simulink model "vasastaden_sort"  (Simulink 5.0)
settings: Solver=FixedStepDiscrete  SolverMode=SingleTasking  StartTime=0  StopTime=Q  FixedStep=1  RelTol=1e-3
values from neighbouring files (symbols this model uses):
  andpt = 1/3    (= 0.333333333333)    [constants_trafik.m]
  andt = 0.1    [constants_trafik.m]
  baseflow = str2num(get(HH, 'String'))    [inputs.m]
  baseflow2 = 0    [areas2.m]
  delayinit = [zeros(1,nr_ex_H2O)]    [constants_trafik.m]
  fast = 0.7    [constants_trafik.m]
  fkmday = in_fkmday    [areas.m]
  fkmday2 = 32067    [areas2.m]
  init_init = 4*3600    (= 14400)    [areas.m]
  init_time = 5    [areas.m]
  K2 = 0.03    [areas2.m]
  nhv = in_nhv/100    [areas.m]
  nhv2 = 5/100    (= 0.05)    [areas2.m]
  nr_ex_H2O = totnr-1    (= 20)    [Prep.m]
  numberOfPersons = in_numberOfPersons    [Prep.m]
  numberOfPersons2 = 5115    [areas2.m]
  othera = in_otherarea    [areas.m]
  othera2 = 42282    [areas2.m]
  othermax = drydepmax*othera    [constants_trafik.m]
  othermax2 = drydepmax*othera2    [areas2.m]
  redu = 0.8    [areas.m]
  roada = in_roads    [areas.m]
  roada2 = 95962    [areas2.m]
  roadaccmax = dryper*24*sph*fast*(p_tyrewear+p_roadwear+p_exhaust+p_breakwear+p_drydep+p_corrZn+p_oildischarge+p_catalyst)    [constants_trafik.m]
  roadaccmax2 = dryper*24*sph*fast*(p_tyrewear2+p_roadwear2+p_exhaust2+p_breakwear2+p_drydep2+p_corrZn2+p_oildischarge2+p_catalyst2)    [areas2.m]
  roadkm = 67e9    (= 67000000000)    [constants_trafik.m]
  roadrunpart = 1    [constants_trafik.m]
  roadwear = 130000    [constants_trafik.m]
  roadZna = in_part_roadZna/100*roada    [areas.m]
  roadZna2 = 2/100*roada2    (= 1919.24)    [areas2.m]
  roofa = in_roofs    [areas.m]
  roofa2 = 92958    [areas2.m]
  RoofCua = in_part_roofCua/100*roofa/cos(15*pi/180)    [areas.m]
  RoofCua2 = 6.9/100*roofa2/cos(15*pi/180)    [areas2.m]
  roofmax = (Znroofmax*RoofZna+Curoofmax*RoofCua)*roofrunpart+drydepmax*roofa    [constants_trafik.m]
  roofmax2 = (Znroofmax*RoofZna2+Curoofmax*RoofCua2)*roofrunpart+drydepmax*roofa2    [areas2.m]
  roofrunpart = 0.7    [constants_trafik.m]
  RoofZna = in_part_roofZna/100*roofa/cos(15*pi/180)    [areas.m]
  RoofZna2 = 6.4/100*roofa2/cos(15*pi/180)    [areas2.m]
  sec_per_ts = in_sec_per_ts    [Prep.m]
  sph = 3600/sec_per_ts    [Prep.m]
  tota = in_tota    [areas.m]
  totnr = 21    [Prep.m]
  tyrewear = 9000    [constants_trafik.m]
  wetdep = [sum(s_wetdep(:,i))]*tota*trans1    [polldistr_gr.m]
  yearly_rain = 1    [Callback_simulate.m]    (also in SEWSYS_fig.m)
undefined symbols (not defined in the file or in its folder): BDT, BODofVS, brakep, catalystp, Curoofp, Drainage, drydep, exhp, Faeces, Industry, K, K2r, oilp, ProcSS_bio, ProcSS_chem, ProcSS_presed, ProcSS_sand, ProcSS_screen, roadp, sani, spBiooxidBod, spBiored, spCcontent, spChemFe, spChemicalPart, spCODBOD, spDenSS, spHeavym, spHjust, spN2ONpurEmitted, spNemitted, spNitrif, spNpur, spOcontent, spPBound, spPout, spPout1, spVSofSS, SSred_bio, SSred_chem, SSred_presed, SSred_sand, SSred_screen, SStoWater, stormw, tyrep, Urine, VSofSS_sand, VSofSS_screen, Znroofp
libraries: SEWSYS_library x1
(part 3 of 3)

== system vasastaden_sort/Separate Sewer System  (1245)/Stormwater/Storm water/Runoff/Subsystem1/if u>0 then u else 1 ==
  note: if u<=0, 0, else u, end
  in_1 : Inport
  Constant : Constant  Value=0
  Switch : Switch  SaturateOnIntegerOverflow=on  InputSameDT=on
  inv. : Fcn  Expr=u
  neg : Gain  Gain=-1  SaturateOnIntegerOverflow=on
  out_1 : Outport  InitialOutput=0
  wires:
  in_1/1 -> inv./1, neg/1
  inv./1 -> Switch/3
  neg/1 -> Switch/2
  Constant/1 -> Switch/1
  Switch/1 -> out_1/1

== system vasastaden_sort/Sewage plant/Biological stage/Predenitri- fication/Nitrification/ denitrification/N-org to NH4/if u>0 then 1/u else 0 ==
  note: if u<=0, 0, else 1/u, end
  in_1 : Inport  Orientation=left
  Constant : Constant  Orientation=left  Value=0
  Constant1 : Constant  Orientation=left
  Switch : Switch  Orientation=left  SaturateOnIntegerOverflow=on  InputSameDT=on
  Switch1 : Switch  Orientation=left  SaturateOnIntegerOverflow=on  InputSameDT=on
  inv. : Fcn  Orientation=left  Expr=1/u
  neg : Gain  Orientation=left  Gain=-1  SaturateOnIntegerOverflow=on
  out_1 : Outport  Orientation=left  InitialOutput=0
  wires:
  Constant1/1 -> Switch1/1
  in_1/1 -> Switch1/3, neg/1
  neg/1 -> Switch1/2, Switch/2
  Switch1/1 -> inv./1
  Switch/1 -> out_1/1
  inv./1 -> Switch/3
  Constant/1 -> Switch/1

== system vasastaden_sort/Separate Sewer System  (36)/Stormwater/Storm water/Add pollutants in rain/Initial loss/Count zeros/Counter1 ==
  Enable : EnablePort  StatesWhenEnabling=reset
  Constant7 : Constant
  Discrete-Time Integrator : DiscreteIntegrator  InitialCondition=1
  Out1 : Outport  InitialOutput=0
  wires:
  Discrete-Time Integrator/1 -> Out1/1
  Constant7/1 -> Discrete-Time Integrator/1

== system vasastaden_sort/Separate Sewer System  (36)/Stormwater/Storm water/Rain -> Stormwater/road surfaces/pollutants on roads/brake wear ==
  note: [ug/fkm]
  Product : Product  Inputs=*/  SaturateOnIntegerOverflow=on  InputSameDT=on
  Product1 : Product  SaturateOnIntegerOverflow=on  InputSameDT=on
  fordonskm/day : Constant  Value=fkmday2
  pollutants from brakes : Constant  Value=brakep
  timesteps/day : Constant  Value=24*sph
  "pollutants [ug) " : Outport
  wires:
  Product1/1 -> "pollutants [ug) "/1
  pollutants from brakes/1 -> Product1/2
  fordonskm/day/1 -> Product/1
  timesteps/day/1 -> Product/2
  Product/1 -> Product1/1

== system vasastaden_sort/Separate Sewer System  (36)/Stormwater/Storm water/Rain -> Stormwater/road surfaces/pollutants on roads/catalyst ==
  note: [ug/fkm]
  Product : Product  Inputs=*/  SaturateOnIntegerOverflow=on  InputSameDT=on
  Product1 : Product  SaturateOnIntegerOverflow=on  InputSameDT=on
  fordonskm/day : Constant  Value=fkmday2
  pollutants from catalysts : Constant  Value=catalystp
  timesteps/day : Constant  Value=24*sph
  "pollutants [ug) " : Outport
  wires:
  Product1/1 -> "pollutants [ug) "/1
  pollutants from catalysts/1 -> Product1/2
  fordonskm/day/1 -> Product/1
  timesteps/day/1 -> Product/2
  Product/1 -> Product1/1

== system vasastaden_sort/Separate Sewer System  (36)/Stormwater/Storm water/Rain -> Stormwater/road surfaces/pollutants on roads/corrosion-Zn ==
  Product : Product  SaturateOnIntegerOverflow=on  InputSameDT=on
  area [m2] : Constant  Value=roadZna2
  avrunnen andel : Gain  Gain=roadrunpart  SaturateOnIntegerOverflow=on
  pollutants from  zink surface : Subsystem
  pollutants [ug] : Outport
  wires:
  Product/1 -> pollutants [ug]/1
  pollutants from  zink surface/1("[ug/m2]") -> avrunnen andel/1
  avrunnen andel/1 -> Product/1
  area [m2]/1 -> Product/2

== system vasastaden_sort/Separate Sewer System  (36)/Stormwater/Storm water/Rain -> Stormwater/road surfaces/pollutants on roads/dry deposition ==
  Product : Product  Inputs=*/  SaturateOnIntegerOverflow=on  InputSameDT=on
  Product1 : Product  SaturateOnIntegerOverflow=on  InputSameDT=on
  area m2 : Constant  Orientation=up  Value=roada2
  timesteps/yr : Constant  Value=365*24*sph
  torrdep ug/m2*yr : Constant  Value=drydep
  pollutants [ug] : Outport
  wires:
  timesteps/yr/1 -> Product/2
  torrdep ug/m2*yr/1 -> Product/1
  Product/1 -> Product1/1
  Product1/1 -> pollutants [ug]/1
  area m2/1 -> Product1/2

== system vasastaden_sort/Separate Sewer System  (36)/Stormwater/Storm water/Rain -> Stormwater/road surfaces/pollutants on roads/exhaust ==
  Product : Product  SaturateOnIntegerOverflow=on  InputSameDT=on
  Product1 : Product  Inputs=*/  SaturateOnIntegerOverflow=on  InputSameDT=on
  fordonskm/day : Constant  Value=fkmday2
  pollutant [ug/fkm] : Constant  Value=exhp
  timesteps/day : Constant  Value=24*sph
  pollutant [ug] : Outport
  wires:
  fordonskm/day/1 -> Product1/1
  timesteps/day/1 -> Product1/2
  Product/1 -> pollutant [ug]/1
  pollutant [ug/fkm]/1 -> Product/2
  Product1/1 -> Product/1

== system vasastaden_sort/Separate Sewer System  (36)/Stormwater/Storm water/Rain -> Stormwater/road surfaces/pollutants on roads/oil discharge ==
  note: [ug/fkm]
  Product : Product  Inputs=*/  SaturateOnIntegerOverflow=on  InputSameDT=on
  Product1 : Product  SaturateOnIntegerOverflow=on  InputSameDT=on
  fordonskm/day : Constant  Value=fkmday2
  pollutants from oil : Constant  Value=oilp
  timesteps/day : Constant  Value=24*sph
  "pollutants [ug) " : Outport
  wires:
  Product/1 -> Product1/1
  timesteps/day/1 -> Product/2
  fordonskm/day/1 -> Product/1
  pollutants from oil/1 -> Product1/2
  Product1/1 -> "pollutants [ug) "/1

== system vasastaden_sort/Separate Sewer System  (36)/Stormwater/Storm water/Rain -> Stormwater/road surfaces/pollutants on roads/road wear ==
  note: kilos of road material
      | per time unit
  Fcn : Fcn  Expr=1-u[1]
  Product : Product  Inputs=3  SaturateOnIntegerOverflow=on  InputSameDT=on
  Product1 : Product  Inputs=3  SaturateOnIntegerOverflow=on  InputSameDT=on
  Product2 : Product  SaturateOnIntegerOverflow=on  InputSameDT=on
  Product3 : Product  Inputs=*/  SaturateOnIntegerOverflow=on  InputSameDT=on
  Road wear : Subsystem
  Sum : Sum  Inputs=|++  SaturateOnIntegerOverflow=on  InputSameDT=on
  andel tunga fordon : Constant  Value=nhv2
  fordonskm/day : Constant  Value=fkmday2
  mg->ug : Gain  Gain=1000  SaturateOnIntegerOverflow=on
  "pollutants in road mat. ppm " : Constant  Orientation=up  Value=roadp
  timesteps/day : Constant  Value=24*sph
  pollutants [ug] : Outport
  wires:
  mg->ug/1 -> pollutants [ug]/1
  Road wear/1(vägslitage kg/tfkm) -> Product/1
  Road wear/2(vägslitage kg/pbkm) -> Product1/3
  Sum/1 -> Product2/1
  Product/1 -> Sum/1
  Product1/1 -> Sum/2
  Fcn/1 -> Product1/2
  andel tunga fordon/1 -> Fcn/1, Product/2
  "pollutants in road mat. ppm "/1 -> Product2/2
  Product2/1 -> mg->ug/1
  timesteps/day/1 -> Product3/2
  fordonskm/day/1 -> Product3/1
  Product3/1 -> Product/3, Product1/1

== system vasastaden_sort/Separate Sewer System  (36)/Stormwater/Storm water/Rain -> Stormwater/road surfaces/pollutants on roads/tyre wear ==
  note: [mg]
  note: Kilos of tyre per
      | time unit
  Fcn : Fcn  Expr=1-u[1]
  Gain : Gain  Gain=1000  SaturateOnIntegerOverflow=on
  Product : Product  Inputs=3  SaturateOnIntegerOverflow=on  InputSameDT=on
  Product1 : Product  Inputs=3  SaturateOnIntegerOverflow=on  InputSameDT=on
  Product2 : Product  SaturateOnIntegerOverflow=on  InputSameDT=on
  Product3 : Product  Inputs=*/  SaturateOnIntegerOverflow=on  InputSameDT=on
  Sum : Sum  Inputs=|++  SaturateOnIntegerOverflow=on  InputSameDT=on
  andel tunga fordon : Constant  Value=nhv2
  fordonskm/day : Constant  Value=fkmday2
  pollutants in tyre  [ppm] : Constant  Orientation=up  Value=tyrep
  timesteps/day : Constant  Value=24*sph
  tyre wear : Subsystem
  pollutants [ug] : Outport
  wires:
  Gain/1 -> pollutants [ug]/1
  pollutants in tyre  [ppm]/1 -> Product2/2
  Sum/1 -> Product2/1
  andel tunga fordon/1 -> Product/2, Fcn/1
  Fcn/1 -> Product1/2
  Product1/1 -> Sum/2
  Product/1 -> Sum/1
  Product2/1 -> Gain/1
  tyre wear/1(tyre wear [kg/tfkm]) -> Product/1
  tyre wear/2(tyre wear [kg/pbkm]) -> Product1/3
  timesteps/day/1 -> Product3/2
  fordonskm/day/1 -> Product3/1
  Product3/1 -> Product/3, Product1/1

== system vasastaden_sort/Separate Sewer System  (36)/Stormwater/Storm water/Rain -> Stormwater/roofs/Pollutants on roofs/Corrosion-Cu ==
  Product : Product  SaturateOnIntegerOverflow=on  InputSameDT=on
  Product1 : Product  Inputs=*/  SaturateOnIntegerOverflow=on  InputSameDT=on
  area [m2] : Constant  Value=RoofCua2
  avrunnen andel : Gain  Gain=roofrunpart  SaturateOnIntegerOverflow=on
  g/m2->ug/m2 : Gain  Gain=1000000  SaturateOnIntegerOverflow=on
  pollutants [g/m2*yr] : Constant  Value=Curoofp
  timesteps/yr : Constant  Value=365*24*sph
  pollutants [ug] : Outport
  wires:
  pollutants [g/m2*yr]/1 -> g/m2->ug/m2/1
  Product1/1 -> avrunnen andel/1
  g/m2->ug/m2/1 -> Product1/1
  timesteps/yr/1 -> Product1/2
  area [m2]/1 -> Product/2
  avrunnen andel/1 -> Product/1
  Product/1 -> pollutants [ug]/1

== system vasastaden_sort/Separate Sewer System  (36)/Stormwater/Storm water/Rain -> Stormwater/roofs/Pollutants on roofs/Corrosion-Zn ==
  Product : Product  SaturateOnIntegerOverflow=on  InputSameDT=on
  Product1 : Product  Inputs=*/  SaturateOnIntegerOverflow=on  InputSameDT=on
  area [m2] : Constant  Value=RoofZna2
  avrunnen andel : Gain  Gain=roofrunpart  SaturateOnIntegerOverflow=on
  g/m2->ug/m2 : Gain  Gain=1000000  SaturateOnIntegerOverflow=on
  pollutants [g/m2*yr] : Constant  Value=Znroofp
  timesteps/yr : Constant  Value=365*24*sph
  pollutants [ug] : Outport
  wires:
  Product1/1 -> avrunnen andel/1
  timesteps/yr/1 -> Product1/2
  pollutants [g/m2*yr]/1 -> g/m2->ug/m2/1
  g/m2->ug/m2/1 -> Product1/1
  Product/1 -> pollutants [ug]/1
  avrunnen andel/1 -> Product/1
  area [m2]/1 -> Product/2

== system vasastaden_sort/Separate Sewer System  (36)/Stormwater/Storm water/Rain -> Stormwater/roofs/Pollutants on roofs/dry deposition ==
  Product : Product  Inputs=*/  SaturateOnIntegerOverflow=on  InputSameDT=on
  Product1 : Product  SaturateOnIntegerOverflow=on  InputSameDT=on
  area m2 : Constant  Orientation=up  Value=roofa2
  timesteps/yr : Constant  Value=365*24*sph
  torrdep ug/m2*yr : Constant  Value=drydep
  pollutants [ug] : Outport
  wires:
  timesteps/yr/1 -> Product/2
  torrdep ug/m2*yr/1 -> Product/1
  Product/1 -> Product1/1
  Product1/1 -> pollutants [ug]/1
  area m2/1 -> Product1/2

== system vasastaden_sort/Separate Sewer System  (1245)/Stormwater/Storm water/Add pollutants in rain/Initial loss/Count zeros/Counter1 ==
  Enable : EnablePort  StatesWhenEnabling=reset
  Constant7 : Constant
  Discrete-Time Integrator : DiscreteIntegrator  InitialCondition=1
  Out1 : Outport  InitialOutput=0
  wires:
  Constant7/1 -> Discrete-Time Integrator/1
  Discrete-Time Integrator/1 -> Out1/1

== system vasastaden_sort/Separate Sewer System  (1245)/Stormwater/Storm water/Rain -> Stormwater/road surfaces/pollutants on roads/brake wear ==
  note: [ug/fkm]
  Product : Product  Inputs=*/  SaturateOnIntegerOverflow=on  InputSameDT=on
  Product1 : Product  SaturateOnIntegerOverflow=on  InputSameDT=on
  fordonskm/day : Constant  Value=fkmday
  pollutants from brakes : Constant  Value=brakep
  timesteps/day : Constant  Value=24*sph
  "pollutants [ug) " : Outport
  wires:
  Product/1 -> Product1/1
  timesteps/day/1 -> Product/2
  fordonskm/day/1 -> Product/1
  pollutants from brakes/1 -> Product1/2
  Product1/1 -> "pollutants [ug) "/1

== system vasastaden_sort/Separate Sewer System  (1245)/Stormwater/Storm water/Rain -> Stormwater/road surfaces/pollutants on roads/catalyst ==
  note: [ug/fkm]
  Product : Product  Inputs=*/  SaturateOnIntegerOverflow=on  InputSameDT=on
  Product1 : Product  SaturateOnIntegerOverflow=on  InputSameDT=on
  fordonskm/day : Constant  Value=fkmday
  pollutants from catalysts : Constant  Value=catalystp
  timesteps/day : Constant  Value=24*sph
  "pollutants [ug) " : Outport
  wires:
  Product/1 -> Product1/1
  timesteps/day/1 -> Product/2
  fordonskm/day/1 -> Product/1
  pollutants from catalysts/1 -> Product1/2
  Product1/1 -> "pollutants [ug) "/1

== system vasastaden_sort/Separate Sewer System  (1245)/Stormwater/Storm water/Rain -> Stormwater/road surfaces/pollutants on roads/corrosion-Zn ==
  Product : Product  SaturateOnIntegerOverflow=on  InputSameDT=on
  area [m2] : Constant  Value=roadZna
  avrunnen andel : Gain  Gain=roadrunpart  SaturateOnIntegerOverflow=on
  pollutants from  zink surface : Subsystem
  pollutants [ug] : Outport
  wires:
  area [m2]/1 -> Product/2
  avrunnen andel/1 -> Product/1
  pollutants from  zink surface/1("[ug/m2]") -> avrunnen andel/1
  Product/1 -> pollutants [ug]/1

== system vasastaden_sort/Separate Sewer System  (1245)/Stormwater/Storm water/Rain -> Stormwater/road surfaces/pollutants on roads/dry deposition ==
  Product : Product  Inputs=*/  SaturateOnIntegerOverflow=on  InputSameDT=on
  Product1 : Product  SaturateOnIntegerOverflow=on  InputSameDT=on
  area m2 : Constant  Orientation=up  Value=roada
  timesteps/yr : Constant  Value=365*24*sph
  torrdep ug/m2*yr : Constant  Value=drydep
  pollutants [ug] : Outport
  wires:
  area m2/1 -> Product1/2
  Product1/1 -> pollutants [ug]/1
  Product/1 -> Product1/1
  torrdep ug/m2*yr/1 -> Product/1
  timesteps/yr/1 -> Product/2

== system vasastaden_sort/Separate Sewer System  (1245)/Stormwater/Storm water/Rain -> Stormwater/road surfaces/pollutants on roads/exhaust ==
  Product : Product  SaturateOnIntegerOverflow=on  InputSameDT=on
  Product1 : Product  Inputs=*/  SaturateOnIntegerOverflow=on  InputSameDT=on
  fordonskm/day : Constant  Value=fkmday
  pollutant [ug/fkm] : Constant  Value=exhp
  timesteps/day : Constant  Value=24*sph
  pollutant [ug] : Outport
  wires:
  Product1/1 -> Product/1
  pollutant [ug/fkm]/1 -> Product/2
  Product/1 -> pollutant [ug]/1
  timesteps/day/1 -> Product1/2
  fordonskm/day/1 -> Product1/1

== system vasastaden_sort/Separate Sewer System  (1245)/Stormwater/Storm water/Rain -> Stormwater/road surfaces/pollutants on roads/oil discharge ==
  note: [ug/fkm]
  Product : Product  Inputs=*/  SaturateOnIntegerOverflow=on  InputSameDT=on
  Product1 : Product  SaturateOnIntegerOverflow=on  InputSameDT=on
  fordonskm/day : Constant  Value=fkmday
  pollutants from oil : Constant  Value=oilp
  timesteps/day : Constant  Value=24*sph
  "pollutants [ug) " : Outport
  wires:
  Product1/1 -> "pollutants [ug) "/1
  pollutants from oil/1 -> Product1/2
  fordonskm/day/1 -> Product/1
  timesteps/day/1 -> Product/2
  Product/1 -> Product1/1

== system vasastaden_sort/Separate Sewer System  (1245)/Stormwater/Storm water/Rain -> Stormwater/road surfaces/pollutants on roads/road wear ==
  note: kilos of road material
      | per time unit
  Fcn : Fcn  Expr=1-u[1]
  Product : Product  Inputs=3  SaturateOnIntegerOverflow=on  InputSameDT=on
  Product1 : Product  Inputs=3  SaturateOnIntegerOverflow=on  InputSameDT=on
  Product2 : Product  SaturateOnIntegerOverflow=on  InputSameDT=on
  Product3 : Product  Inputs=*/  SaturateOnIntegerOverflow=on  InputSameDT=on
  Road wear : Subsystem
  Sum : Sum  Inputs=|++  SaturateOnIntegerOverflow=on  InputSameDT=on
  andel tunga fordon : Constant  Value=nhv
  fordonskm/day : Constant  Value=fkmday
  mg->ug : Gain  Gain=1000  SaturateOnIntegerOverflow=on
  "pollutants in road mat. ppm " : Constant  Orientation=up  Value=roadp
  timesteps/day : Constant  Value=24*sph
  pollutants [ug] : Outport
  wires:
  Product3/1 -> Product1/1, Product/3
  fordonskm/day/1 -> Product3/1
  timesteps/day/1 -> Product3/2
  Product2/1 -> mg->ug/1
  "pollutants in road mat. ppm "/1 -> Product2/2
  andel tunga fordon/1 -> Product/2, Fcn/1
  Fcn/1 -> Product1/2
  Product1/1 -> Sum/2
  Product/1 -> Sum/1
  Sum/1 -> Product2/1
  Road wear/2(vägslitage kg/pbkm) -> Product1/3
  Road wear/1(vägslitage kg/tfkm) -> Product/1
  mg->ug/1 -> pollutants [ug]/1

== system vasastaden_sort/Separate Sewer System  (1245)/Stormwater/Storm water/Rain -> Stormwater/road surfaces/pollutants on roads/tyre wear ==
  note: Kilos of tyre per
      | time unit
  note: [mg]
  Fcn : Fcn  Expr=1-u[1]
  Gain : Gain  Gain=1000  SaturateOnIntegerOverflow=on
  Product : Product  Inputs=3  SaturateOnIntegerOverflow=on  InputSameDT=on
  Product1 : Product  Inputs=3  SaturateOnIntegerOverflow=on  InputSameDT=on
  Product2 : Product  SaturateOnIntegerOverflow=on  InputSameDT=on
  Product3 : Product  Inputs=*/  SaturateOnIntegerOverflow=on  InputSameDT=on
  Sum : Sum  Inputs=|++  SaturateOnIntegerOverflow=on  InputSameDT=on
  andel tunga fordon : Constant  Value=nhv
  fordonskm/day : Constant  Value=fkmday
  pollutants in tyre  [ppm] : Constant  Orientation=up  Value=tyrep
  timesteps/day : Constant  Value=24*sph
  tyre wear : Subsystem
  pollutants [ug] : Outport
  wires:
  Product3/1 -> Product1/1, Product/3
  fordonskm/day/1 -> Product3/1
  timesteps/day/1 -> Product3/2
  tyre wear/2(tyre wear [kg/pbkm]) -> Product1/3
  tyre wear/1(tyre wear [kg/tfkm]) -> Product/1
  Product2/1 -> Gain/1
  Product/1 -> Sum/1
  Product1/1 -> Sum/2
  Fcn/1 -> Product1/2
  andel tunga fordon/1 -> Fcn/1, Product/2
  Sum/1 -> Product2/1
  pollutants in tyre  [ppm]/1 -> Product2/2
  Gain/1 -> pollutants [ug]/1

== system vasastaden_sort/Separate Sewer System  (1245)/Stormwater/Storm water/Rain -> Stormwater/roofs/Pollutants on roofs/Corrosion-Cu ==
  Product : Product  SaturateOnIntegerOverflow=on  InputSameDT=on
  Product1 : Product  Inputs=*/  SaturateOnIntegerOverflow=on  InputSameDT=on
  area [m2] : Constant  Value=RoofCua
  avrunnen andel : Gain  Gain=roofrunpart  SaturateOnIntegerOverflow=on
  g/m2->ug/m2 : Gain  Gain=1000000  SaturateOnIntegerOverflow=on
  pollutants [g/m2*yr] : Constant  Value=Curoofp
  timesteps/yr : Constant  Value=365*24*sph
  pollutants [ug] : Outport
  wires:
  Product/1 -> pollutants [ug]/1
  avrunnen andel/1 -> Product/1
  area [m2]/1 -> Product/2
  timesteps/yr/1 -> Product1/2
  g/m2->ug/m2/1 -> Product1/1
  Product1/1 -> avrunnen andel/1
  pollutants [g/m2*yr]/1 -> g/m2->ug/m2/1

== system vasastaden_sort/Separate Sewer System  (1245)/Stormwater/Storm water/Rain -> Stormwater/roofs/Pollutants on roofs/Corrosion-Zn ==
  Product : Product  SaturateOnIntegerOverflow=on  InputSameDT=on
  Product1 : Product  Inputs=*/  SaturateOnIntegerOverflow=on  InputSameDT=on
  area [m2] : Constant  Value=RoofZna
  avrunnen andel : Gain  Gain=roofrunpart  SaturateOnIntegerOverflow=on
  g/m2->ug/m2 : Gain  Gain=1000000  SaturateOnIntegerOverflow=on
  pollutants [g/m2*yr] : Constant  Value=Znroofp
  timesteps/yr : Constant  Value=365*24*sph
  pollutants [ug] : Outport
  wires:
  area [m2]/1 -> Product/2
  avrunnen andel/1 -> Product/1
  Product/1 -> pollutants [ug]/1
  g/m2->ug/m2/1 -> Product1/1
  pollutants [g/m2*yr]/1 -> g/m2->ug/m2/1
  timesteps/yr/1 -> Product1/2
  Product1/1 -> avrunnen andel/1

== system vasastaden_sort/Separate Sewer System  (1245)/Stormwater/Storm water/Rain -> Stormwater/roofs/Pollutants on roofs/dry deposition ==
  Product : Product  Inputs=*/  SaturateOnIntegerOverflow=on  InputSameDT=on
  Product1 : Product  SaturateOnIntegerOverflow=on  InputSameDT=on
  area m2 : Constant  Orientation=up  Value=roofa
  timesteps/yr : Constant  Value=365*24*sph
  torrdep ug/m2*yr : Constant  Value=drydep
  pollutants [ug] : Outport
  wires:
  area m2/1 -> Product1/2
  Product1/1 -> pollutants [ug]/1
  Product/1 -> Product1/1
  torrdep ug/m2*yr/1 -> Product/1
  timesteps/yr/1 -> Product/2

== system vasastaden_sort/Separate Sewer System  (36)/Stormwater/Storm water/Rain -> Stormwater/road surfaces/pollutants on roads/corrosion-Zn/pollutants from  zink surface ==
  Product : Product  Inputs=*/  SaturateOnIntegerOverflow=on  InputSameDT=on
  g/m2->ug/m2 : Gain  Gain=1000000  SaturateOnIntegerOverflow=on
  pollutants [g/m2*yr] : Constant  Value=Znroofp
  timesteps/yr : Constant  Value=365*24*sph
  "[ug/m2]" : Outport
  wires:
  Product/1 -> "[ug/m2]"/1
  timesteps/yr/1 -> Product/2
  pollutants [g/m2*yr]/1 -> g/m2->ug/m2/1
  g/m2->ug/m2/1 -> Product/1

== system vasastaden_sort/Separate Sewer System  (36)/Stormwater/Storm water/Rain -> Stormwater/road surfaces/pollutants on roads/road wear/Road wear ==
  Constant : Constant  Value=[andt roadkm roadwear andpt]
  Fcn : Fcn  Expr=(u[3]*u[4])/(u[1]*u[2])
  Fcn1 : Fcn  Expr=(u[3]*(1-u[4]))/(u[2]*(1-u[1]))
  Gain : Gain  Gain=[1 1 1000 1]  SaturateOnIntegerOverflow=on
  vägslitage kg/tfkm : Outport
  vägslitage kg/pbkm : Outport  Port=2
  wires:
  Gain/1 -> Fcn1/1, Fcn/1
  Constant/1 -> Gain/1
  Fcn/1 -> vägslitage kg/tfkm/1
  Fcn1/1 -> vägslitage kg/pbkm/1

== system vasastaden_sort/Separate Sewer System  (36)/Stormwater/Storm water/Rain -> Stormwater/road surfaces/pollutants on roads/tyre wear/tyre wear ==
  note: change of units
      | tons-kg
  Constant : Constant  Value=[andt roadkm tyrewear andpt]
  Fcn : Fcn  Expr=(u[3]*u[4])/(u[1]*u[2])
  Fcn1 : Fcn  Expr=(u[3]*(1-u[4]))/(u[2]*(1-u[1]))
  Gain : Gain  Gain=[1 1 1000 1]  SaturateOnIntegerOverflow=on
  tyre wear [kg/tfkm] : Outport
  tyre wear [kg/pbkm] : Outport  Port=2
  wires:
  Gain/1 -> Fcn1/1, Fcn/1
  Constant/1 -> Gain/1
  Fcn/1 -> tyre wear [kg/tfkm]/1
  Fcn1/1 -> tyre wear [kg/pbkm]/1

== system vasastaden_sort/Separate Sewer System  (1245)/Stormwater/Storm water/Rain -> Stormwater/road surfaces/pollutants on roads/corrosion-Zn/pollutants from  zink surface ==
  Product : Product  Inputs=*/  SaturateOnIntegerOverflow=on  InputSameDT=on
  g/m2->ug/m2 : Gain  Gain=1000000  SaturateOnIntegerOverflow=on
  pollutants [g/m2*yr] : Constant  Value=Znroofp
  timesteps/yr : Constant  Value=365*24*sph
  "[ug/m2]" : Outport
  wires:
  g/m2->ug/m2/1 -> Product/1
  pollutants [g/m2*yr]/1 -> g/m2->ug/m2/1
  timesteps/yr/1 -> Product/2
  Product/1 -> "[ug/m2]"/1

== system vasastaden_sort/Separate Sewer System  (1245)/Stormwater/Storm water/Rain -> Stormwater/road surfaces/pollutants on roads/road wear/Road wear ==
  Constant : Constant  Value=[andt roadkm roadwear andpt]
  Fcn : Fcn  Expr=(u[3]*u[4])/(u[1]*u[2])
  Fcn1 : Fcn  Expr=(u[3]*(1-u[4]))/(u[2]*(1-u[1]))
  Gain : Gain  Gain=[1 1 1000 1]  SaturateOnIntegerOverflow=on
  vägslitage kg/tfkm : Outport
  vägslitage kg/pbkm : Outport  Port=2
  wires:
  Fcn1/1 -> vägslitage kg/pbkm/1
  Fcn/1 -> vägslitage kg/tfkm/1
  Constant/1 -> Gain/1
  Gain/1 -> Fcn/1, Fcn1/1

== system vasastaden_sort/Separate Sewer System  (1245)/Stormwater/Storm water/Rain -> Stormwater/road surfaces/pollutants on roads/tyre wear/tyre wear ==
  note: change of units
      | tons-kg
  Constant : Constant  Value=[andt roadkm tyrewear andpt]
  Fcn : Fcn  Expr=(u[3]*u[4])/(u[1]*u[2])
  Fcn1 : Fcn  Expr=(u[3]*(1-u[4]))/(u[2]*(1-u[1]))
  Gain : Gain  Gain=[1 1 1000 1]  SaturateOnIntegerOverflow=on
  tyre wear [kg/tfkm] : Outport
  tyre wear [kg/pbkm] : Outport  Port=2
  wires:
  Fcn1/1 -> tyre wear [kg/pbkm]/1
  Fcn/1 -> tyre wear [kg/tfkm]/1
  Constant/1 -> Gain/1
  Gain/1 -> Fcn/1, Fcn1/1
